simulink model "controllo_PI_sim"  (R2020b)
settings: Solver=VariableStepAuto  StartTime=0.0  StopTime=20  RelTol=1e-3
libraries: cstblocks x3
settings Model: Creator=miche  LastModifiedBy=miche

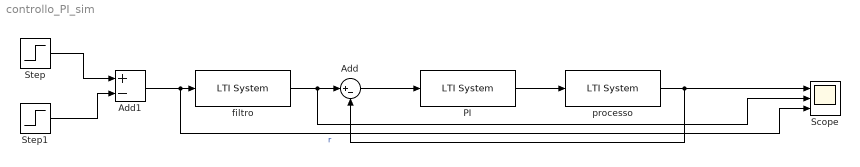
== system controllo_PI_sim ==
  Add : Sum  Inputs=|+-
  Add1 : Sum  Inputs=+-
  PI : cstblocks/LTI System  sys=C  IC=[]
  Scope : Scope  NumInputPorts=3
  Step : Step  Time=0  After=3  SampleTime=0
  Step1 : Step  Time=10  After=2  SampleTime=0
  filtro : cstblocks/LTI System  sys=F  IC=[]
  processo : cstblocks/LTI System  sys=P  IC=[]
  wires:
  PI/1 -> processo/1
  processo/1 -> Scope/1, Add/2
  Add/1 -> PI/1
  Step/1 -> Add1/1
  Add1/1 -> Scope/3, filtro/1  "r"
  Step1/1 -> Add1/2
  filtro/1 -> Scope/2, Add/1
